simulink model "Foc"  (R2025b)
settings: Solver=FixedStepDiscrete  StartTime=0.0  StopTime=10.0  FixedStep=0.001  RelTol=1e-3
values from neighbouring files (symbols this model uses):
  cal_bActHwMode = NoneSAR.Parameter    [Foc_2024b_LoadCalParameter.m]    (also in Foc_LoadCalParameter.m)
  cal_f32AdcMaxCountsHw = NoneSAR.Parameter    [Foc_LoadCalParameter.m]
  cal_f32AdcRefVoltHw = NoneSAR.Parameter    [Foc_LoadCalParameter.m]
  cal_f32AdcVoltMidHw = NoneSAR.Parameter    [Foc_LoadCalParameter.m]
  cal_f32FullScaleCur = NoneSAR.Parameter    [Foc_LoadCalParameter.m]
  cal_f32GainAmpHw = NoneSAR.Parameter    [Foc_LoadCalParameter.m]
  cal_f32OhmRShuntHw = NoneSAR.Parameter    [Foc_LoadCalParameter.m]
  cal_s16HwtDutyU = NoneSAR.Parameter    [Foc_LoadCalParameter.m]
  cal_s16HwtDutyV = NoneSAR.Parameter    [Foc_LoadCalParameter.m]
  cal_s16HwtDutyW = NoneSAR.Parameter    [Foc_LoadCalParameter.m]
  cal_s16IdKi = NoneSAR.Parameter    [Foc_LoadCalParameter.m]
  cal_s16IdKp = NoneSAR.Parameter    [Foc_LoadCalParameter.m]
  cal_s16IdMaxOut = NoneSAR.Parameter    [Foc_LoadCalParameter.m]
  cal_s16IdMinOut = NoneSAR.Parameter    [Foc_LoadCalParameter.m]
  cal_s16Inductivity = NoneSAR.Parameter    [Foc_2024b_LoadCalParameter.m]    (also in Foc_LoadCalParameter.m)
  cal_s16IqKi = NoneSAR.Parameter    [Foc_LoadCalParameter.m]
  cal_s16IqKp = NoneSAR.Parameter    [Foc_LoadCalParameter.m]
  cal_s16IqMaxOut = NoneSAR.Parameter    [Foc_LoadCalParameter.m]
  cal_s16IqMinOut = NoneSAR.Parameter    [Foc_LoadCalParameter.m]
  cal_s16LpfPllEst = NoneSAR.Parameter    [Foc_2024b_LoadCalParameter.m]    (also in Foc_LoadCalParameter.m)
  cal_s16LpfPllEstOpenLoop = NoneSAR.Parameter    [Foc_2024b_LoadCalParameter.m]    (also in Foc_LoadCalParameter.m)
  cal_s16MinSampleTime = NoneSAR.Parameter    [Foc_2024b_LoadCalParameter.m]    (also in Foc_LoadCalParameter.m)
  cal_s16OmegaGainEst = NoneSAR.Parameter    [Foc_2024b_LoadCalParameter.m]    (also in Foc_LoadCalParameter.m)
  cal_s16RPha = NoneSAR.Parameter    [Foc_2024b_LoadCalParameter.m]    (also in Foc_LoadCalParameter.m)
  cal_s16ThresholdPhaCurImplaisible = NoneSAR.Parameter    [Foc_2024b_LoadCalParameter.m]    (also in Foc_LoadCalParameter.m)
  cal_s8IdFacKi = NoneSAR.Parameter    [Foc_LoadCalParameter.m]
  cal_s8IdFacKp = NoneSAR.Parameter    [Foc_LoadCalParameter.m]
  cal_s8IqFacKi = NoneSAR.Parameter    [Foc_LoadCalParameter.m]
  cal_s8IqFacKp = NoneSAR.Parameter    [Foc_LoadCalParameter.m]
  cal_u16AdcTriggerOffset = NoneSAR.Parameter    [Foc_LoadCalParameter.m]
  cal_u8HwtSector = NoneSAR.Parameter    [Foc_LoadCalParameter.m]
  cal_u8TiDebPhaCur = NoneSAR.Parameter    [Foc_2024b_LoadCalParameter.m]    (also in Foc_LoadCalParameter.m)
undefined symbols (not defined in the file or in its folder): CCU6_T12PERIOD, CCU_PWM_PERIOD_TICKS_HALF, DCLINK_VOLTAGE_FACTOR, DesiredPwm_U, DesiredPwm_V, DesiredPwm_W, e_motorstate_t, e_running_dir_t, FOC_SVM_MAX, FOC_VD_VQ_MAX, FOC_VD_VQ_MAX_100, FOC_VD_VQ_MAX_95, FOC_VD_VQ_MAX_97, FOCLLD_CCU_PWM_PERIOD_TICKS_HALF, FOCLLD_SKIP_DEAD_TIME_THRESHOLD, MAX_DUTY, MIN_SAMPLE_TIME_DEFAULT, MODULATION_FLATBOTTOM, ONEBY_CURRENT_AMPLIFICATION, PhaseCurrentU, PhaseCurrentV, PhaseCurrentW, PwmShift_DutyLong, PwmShift_DutyMed, PwmShift_DutyShort, PwmShiftPtr_RiseLong, PwmShiftPtr_RiseMed, PwmShiftPtr_RiseShort, s16_EST_THETA_GAIN, s16_ONEBYSQR3, s16_SQR3OVER2, st_c_pi_Q_s16_outMax, st_c_pi_Q_s16_outMin, U8_INDUCTIVITY_FAC, VQ_MAX_TABLE_SIZE, VqMaxTable_100, VqMaxTable_95, VqMaxTable_97
libraries: simulink x16, hdlsllib x2
(part 5 of 6)

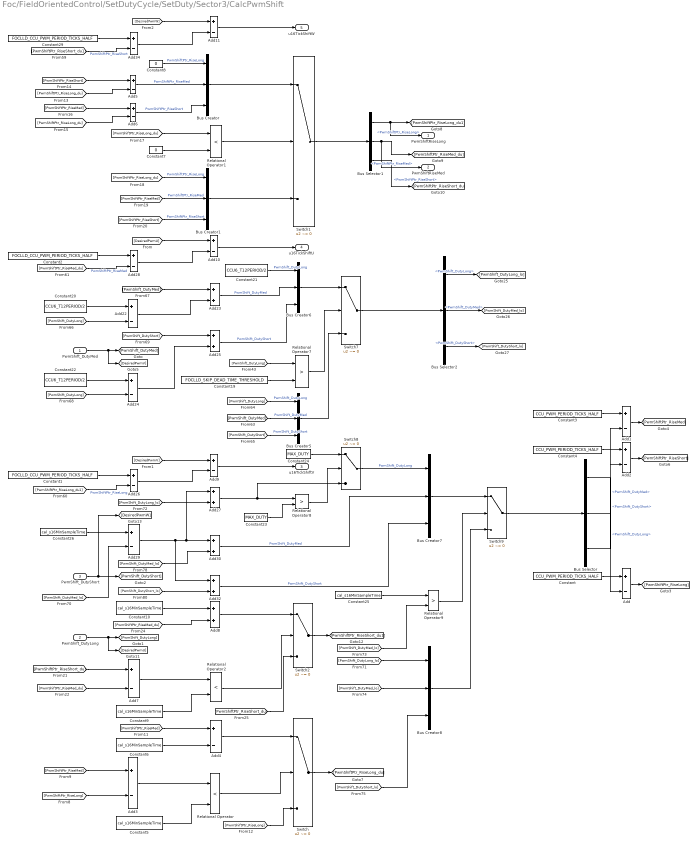
== system Foc/FieldOrientedControl/SetDutyCycle/SetDuty/Sector3/CalcPwmShift ==
  PwmShift_DutyMed : Inport
  PwmShift_DutyLong : Inport  Port=2
  PwmShift_DutyShort : Inport  Port=3
  Add{,1..7,9..11,22,24,26,28..29,34} (17 alike) : Sum  Inputs=+-
  Add{8,23,25,27,30,32} (6 alike) : Sum
  Bus Creator : BusCreator  Inputs=PwmShiftPtr_RiseLong,PwmShiftPtr_RiseMed,PwmShiftPtr_RiseShort
  Bus Creator1 : BusCreator  Inputs=PwmShiftPtr_RiseLong,PwmShiftPtr_RiseMed,PwmShiftPtr_RiseShort
  Bus Creator{5..8} (4 alike) : BusCreator  Inputs=PwmShift_DutyLong,PwmShift_DutyMed,PwmShift_DutyShort
  Bus Selector : BusSelector  OutputSignals=PwmShift_DutyLong,PwmShift_DutyMed,PwmShift_DutyShort
  Bus Selector1 : BusSelector  OutputSignals=PwmShiftPtr_RiseLong,PwmShiftPtr_RiseMed,PwmShiftPtr_RiseShort
  Bus Selector2 : BusSelector  OutputSignals=PwmShift_DutyLong,PwmShift_DutyMed,PwmShift_DutyShort
  Constant : Constant  Value=CCU_PWM_PERIOD_TICKS_HALF
  Constant1 : Constant  Value=FOCLLD_CCU_PWM_PERIOD_TICKS_HALF
  Constant{5..6,9..10,25..26} (6 alike) : Constant  Value=cal_s16MinSampleTime
  Constant19 : Constant  Value=FOCLLD_SKIP_DEAD_TIME_THRESHOLD
  Constant2 : Constant  Value=FOCLLD_CCU_PWM_PERIOD_TICKS_HALF
  Constant20 : Constant  Value=CCU6_T12PERIOD/2
  Constant21 : Constant  Value=CCU6_T12PERIOD/2
  Constant22 : Constant  Value=CCU6_T12PERIOD/2
  Constant23 : Constant  Value=MAX_DUTY
  Constant24 : Constant  Value=MAX_DUTY
  Constant29 : Constant  Value=FOCLLD_CCU_PWM_PERIOD_TICKS_HALF
  Constant3 : Constant  Value=CCU_PWM_PERIOD_TICKS_HALF
  Constant4 : Constant  Value=CCU_PWM_PERIOD_TICKS_HALF
  Constant7 : Constant  Value=0  OutDataTypeStr=int16
  Constant8 : Constant  Value=0  OutDataTypeStr=int16
  Relational Operator : RelationalOperator  Operator=<  OutDataTypeStr=boolean  RndMeth=Simplest  InputSameDT=off
  Relational Operator1 : RelationalOperator  Operator=<  OutDataTypeStr=boolean  RndMeth=Simplest  InputSameDT=off
  Relational Operator2 : RelationalOperator  Operator=<  OutDataTypeStr=boolean  RndMeth=Simplest  InputSameDT=off
  Relational Operator7 : RelationalOperator  Operator=>  OutDataTypeStr=boolean  RndMeth=Simplest  InputSameDT=off
  Relational Operator8 : RelationalOperator  Operator=>  OutDataTypeStr=boolean  RndMeth=Simplest  InputSameDT=off
  Relational Operator9 : RelationalOperator  Operator=>  OutDataTypeStr=boolean  RndMeth=Simplest  InputSameDT=off
  Switch{,1..2,7..9} (6 alike) : Switch  Criteria=u2 ~= 0  SaturateOnIntegerOverflow=off  InputSameDT=off
  PwmShiftRiseLong : Outport
  PwmShiftRiseMed : Outport  Port=2
  u16TickShiftV : Outport  Port=3  OutDataTypeStr=uint16
  u16TickShiftU : Outport  Port=4  OutDataTypeStr=uint16
  u16TickShiftW : Outport  Port=5  OutDataTypeStr=uint16
  wires:
  Constant2/1 -> Add28/1
  [PwmShiftPtr_RiseLong_du] -> Add5/2
  Constant29/1 -> Add34/1
  [PwmShiftPtr_RiseShort_du1] -> Add34/2  "PwmShiftPtr_RiseShort"
  Bus Creator/1 -> Switch1/1
  [PwmShiftPtr_RiseShort] -> Add5/1
  [PwmShiftPtr_RiseMed] -> Add6/1
  [PwmShiftPtr_RiseLong_du] -> Add6/2
  [PwmShiftPtr_RiseMed_du] -> Add28/2  "PwmShiftPtr_RiseMed"
  Constant20/1 -> Add22/1
  [PwmShift_DutyLong] -> Add22/2
  PwmShift_DutyMed/1 -> [DesiredPwmV], [PwmShift_DutyMed]
  Constant22/1 -> Add24/1
  Relational Operator1/1 -> Switch1/2
  [PwmShift_DutyLong] -> Add24/2
  Constant1/1 -> Add26/1
  [PwmShiftPtr_RiseLong_du1] -> Add26/2  "PwmShiftPtr_RiseLong"
  Add7/1 -> Relational Operator2/1
  Constant26/1 -> Add29/1
  PwmShift_DutyShort/1 -> [DesiredPwmW], [PwmShift_DutyShort]
  Bus Creator7/1 -> Switch9/1
  [PwmShift_DutyMed_lo] -> Add29/2
  PwmShift_DutyLong/1 -> [DesiredPwmU], [PwmShift_DutyLong]
  Add22/1 -> Add23/2
  Add8/1 -> Switch2/1
  [PwmShiftPtr_RiseShort_du] -> Add7/1
  [PwmShiftPtr_RiseMed_du] -> Add7/2
  Bus Selector2/2 -> [PwmShift_DutyMed_lo]  "<PwmShift_DutyMed>"
  [PwmShiftPtr_RiseMed] -> Add3/1
  Add29/1 -> Add30/1, Add27/1, Add32/1
  [PwmShiftPtr_RiseLong] -> Add3/2
  [DesiredPwmW] -> Add11/1
  Add34/1 -> Add11/2
  Constant8/1 -> Bus Creator/1  "PwmShiftPtr_RiseLong"
  Add10/1 -> u16TickShiftU/1
  Add5/1 -> Bus Creator/2  "PwmShiftPtr_RiseMed"
  [PwmShiftPtr_RiseMed_du] -> Add8/2
  Add11/1 -> u16TickShiftW/1
  Add6/1 -> Bus Creator/3  "PwmShiftPtr_RiseShort"
  [PwmShiftPtr_RiseLong_du] -> Relational Operator1/1
  Constant7/1 -> Relational Operator1/2
  [PwmShiftPtr_RiseLong_du] -> Bus Creator1/1  "PwmShiftPtr_RiseLong"
  [PwmShiftPtr_RiseMed] -> Bus Creator1/2  "PwmShiftPtr_RiseMed"
  [PwmShiftPtr_RiseShort] -> Bus Creator1/3  "PwmShiftPtr_RiseShort"
  [DesiredPwmU] -> Add10/1
  [PwmShift_DutyMed] -> Add23/1
  Add28/1 -> Add10/2
  Add25/1 -> Bus Creator6/3  "PwmShift_DutyShort"
  [PwmShift_DutyShort] -> Add25/1
  [PwmShift_DutyLong] -> Relational Operator7/1
  Add24/1 -> Add25/2
  [DesiredPwmV] -> Add9/1
  Add26/1 -> Add9/2
  [PwmShift_DutyLong_lo] -> Add27/2
  Bus Selector1/1 -> PwmShiftRiseLong/1, [PwmShiftPtr_RiseLong_du1]  "<PwmShiftPtr_RiseLong>"
  [PwmShift_DutyMed_lo] -> Add30/2
  [PwmShift_DutyShort_lo] -> Add32/2
  Constant10/1 -> Add8/1
  Constant9/1 -> Relational Operator2/2
  [PwmShiftPtr_RiseMed] -> Add4/1
  Constant6/1 -> Add4/2
  Add3/1 -> Relational Operator/1
  Constant5/1 -> Relational Operator/2
  Bus Creator1/1 -> Switch1/3
  Constant21/1 -> Bus Creator6/1  "PwmShift_DutyLong"
  Add23/1 -> Bus Creator6/2  "PwmShift_DutyMed"
  Constant19/1 -> Relational Operator7/2
  [PwmShift_DutyLong] -> Bus Creator5/1  "PwmShift_DutyLong"
  [PwmShift_DutyMed] -> Bus Creator5/2  "PwmShift_DutyMed"
  Add9/1 -> u16TickShiftV/1
  [PwmShift_DutyShort] -> Bus Creator5/3  "PwmShift_DutyShort"
  Add27/1 -> Switch8/3, Relational Operator8/1
  Constant23/1 -> Relational Operator8/2
  Add30/1 -> Bus Creator7/2  "PwmShift_DutyMed"
  Add32/1 -> Bus Creator7/3  "PwmShift_DutyShort"
  Relational Operator2/1 -> Switch2/2
  [PwmShiftPtr_RiseShort_du] -> Switch2/3
  Add4/1 -> Switch/1
  Relational Operator/1 -> Switch/2
  [PwmShiftPtr_RiseLong] -> Switch/3
  Switch1/1 -> Bus Selector1/1
  Bus Creator6/1 -> Switch7/1
  Relational Operator7/1 -> Switch7/2
  [PwmShift_DutyMed_lo] -> Relational Operator9/2
  Bus Creator5/1 -> Switch7/3
  Constant24/1 -> Switch8/1
  Relational Operator8/1 -> Switch8/2
  Switch2/1 -> [PwmShiftPtr_RiseShort_du1]
  Switch/1 -> [PwmShiftPtr_RiseLong_du]
  Bus Selector1/2 -> PwmShiftRiseMed/1, [PwmShiftPtr_RiseMed_du]  "<PwmShiftPtr_RiseMed>"
  Bus Selector1/3 -> [PwmShiftPtr_RiseShort_du]  "<PwmShiftPtr_RiseShort>"
  Switch7/1 -> Bus Selector2/1
  Switch8/1 -> Bus Creator7/1  "PwmShift_DutyLong"
  Constant25/1 -> Relational Operator9/1
  [PwmShift_DutyLong_lo] -> Bus Creator8/1
  Bus Selector/2 -> Add1/2  "<PwmShift_DutyMed>"
  [PwmShift_DutyMed_lo] -> Bus Creator8/2
  [PwmShift_DutyShort_lo] -> Bus Creator8/3
  Bus Selector2/1 -> [PwmShift_DutyLong_lo]  "<PwmShift_DutyLong>"
  Bus Selector2/3 -> [PwmShift_DutyShort_lo]  "<PwmShift_DutyShort>"
  Relational Operator9/1 -> Switch9/2
  Bus Creator8/1 -> Switch9/3
  Switch9/1 -> Bus Selector/1
  Constant3/1 -> Add1/1
  Constant4/1 -> Add2/1
  Bus Selector/1 -> Add/2  "<PwmShift_DutyLong>"
  Bus Selector/3 -> Add2/2  "<PwmShift_DutyShort>"
  Constant/1 -> Add/1
  Add1/1 -> [PwmShiftPtr_RiseMed]
  Add2/1 -> [PwmShiftPtr_RiseShort]
  Add/1 -> [PwmShiftPtr_RiseLong]

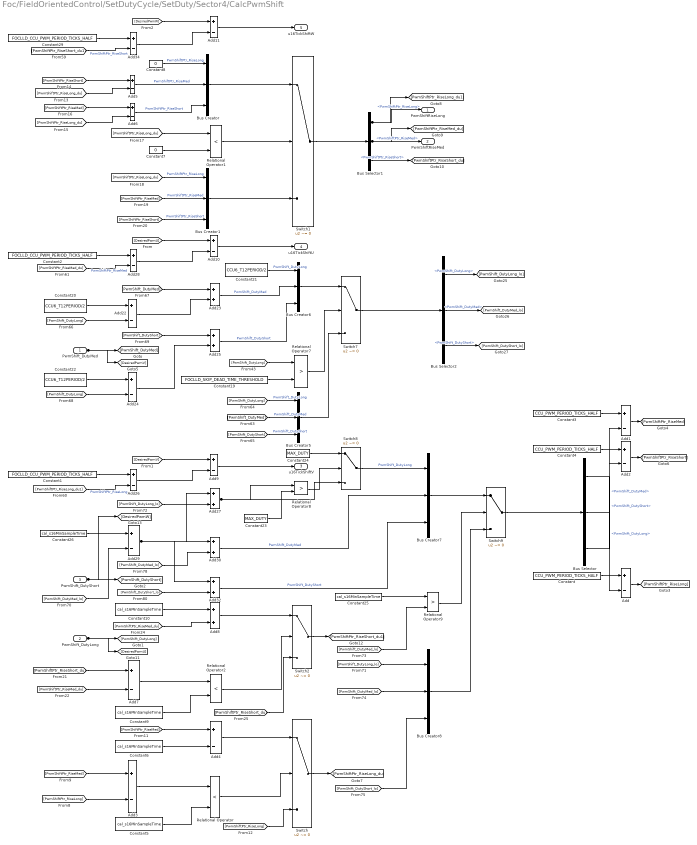
== system Foc/FieldOrientedControl/SetDutyCycle/SetDuty/Sector4/CalcPwmShift ==
  PwmShift_DutyMed : Inport
  PwmShift_DutyLong : Inport  Port=2
  PwmShift_DutyShort : Inport  Port=3
  Add{,1..7,9..11,22,24,26,28..29,34} (17 alike) : Sum  Inputs=+-
  Add{8,23,25,27,30,32} (6 alike) : Sum
  Bus Creator : BusCreator  Inputs=PwmShiftPtr_RiseLong,PwmShiftPtr_RiseMed,PwmShiftPtr_RiseShort
  Bus Creator1 : BusCreator  Inputs=PwmShiftPtr_RiseLong,PwmShiftPtr_RiseMed,PwmShiftPtr_RiseShort
  Bus Creator{5..8} (4 alike) : BusCreator  Inputs=PwmShift_DutyLong,PwmShift_DutyMed,PwmShift_DutyShort
  Bus Selector : BusSelector  OutputSignals=PwmShift_DutyLong,PwmShift_DutyMed,PwmShift_DutyShort
  Bus Selector1 : BusSelector  OutputSignals=PwmShiftPtr_RiseLong,PwmShiftPtr_RiseMed,PwmShiftPtr_RiseShort
  Bus Selector2 : BusSelector  OutputSignals=PwmShift_DutyLong,PwmShift_DutyMed,PwmShift_DutyShort
  Constant : Constant  Value=CCU_PWM_PERIOD_TICKS_HALF
  Constant1 : Constant  Value=FOCLLD_CCU_PWM_PERIOD_TICKS_HALF
  Constant{5..6,9..10,25..26} (6 alike) : Constant  Value=cal_s16MinSampleTime
  Constant19 : Constant  Value=FOCLLD_SKIP_DEAD_TIME_THRESHOLD
  Constant2 : Constant  Value=FOCLLD_CCU_PWM_PERIOD_TICKS_HALF
  Constant20 : Constant  Value=CCU6_T12PERIOD/2
  Constant21 : Constant  Value=CCU6_T12PERIOD/2
  Constant22 : Constant  Value=CCU6_T12PERIOD/2
  Constant23 : Constant  Value=MAX_DUTY
  Constant24 : Constant  Value=MAX_DUTY
  Constant29 : Constant  Value=FOCLLD_CCU_PWM_PERIOD_TICKS_HALF
  Constant3 : Constant  Value=CCU_PWM_PERIOD_TICKS_HALF
  Constant4 : Constant  Value=CCU_PWM_PERIOD_TICKS_HALF
  Constant7 : Constant  Value=0  OutDataTypeStr=int16
  Constant8 : Constant  Value=0  OutDataTypeStr=int16
  Relational Operator : RelationalOperator  Operator=<  OutDataTypeStr=boolean  RndMeth=Simplest  InputSameDT=off
  Relational Operator1 : RelationalOperator  Operator=<  OutDataTypeStr=boolean  RndMeth=Simplest  InputSameDT=off
  Relational Operator2 : RelationalOperator  Operator=<  OutDataTypeStr=boolean  RndMeth=Simplest  InputSameDT=off
  Relational Operator7 : RelationalOperator  Operator=>  OutDataTypeStr=boolean  RndMeth=Simplest  InputSameDT=off
  Relational Operator8 : RelationalOperator  Operator=>  OutDataTypeStr=boolean  RndMeth=Simplest  InputSameDT=off
  Relational Operator9 : RelationalOperator  Operator=>  OutDataTypeStr=boolean  RndMeth=Simplest  InputSameDT=off
  Switch{,1..2,7..9} (6 alike) : Switch  Criteria=u2 ~= 0  SaturateOnIntegerOverflow=off  InputSameDT=off
  PwmShiftRiseLong : Outport
  PwmShiftRiseMed : Outport  Port=2
  u16TickShiftV : Outport  Port=3  OutDataTypeStr=uint16
  u16TickShiftU : Outport  Port=4  OutDataTypeStr=uint16
  u16TickShiftW : Outport  Port=5  OutDataTypeStr=uint16
  wires:
  Constant2/1 -> Add28/1
  [PwmShiftPtr_RiseLong_du] -> Add5/2
  Constant29/1 -> Add34/1
  [PwmShiftPtr_RiseLong_du] -> Add6/2
  [PwmShiftPtr_RiseShort_du1] -> Add34/2  "PwmShiftPtr_RiseShort"
  Bus Creator/1 -> Switch1/1
  [PwmShiftPtr_RiseShort] -> Add5/1
  Add10/1 -> u16TickShiftU/1
  [PwmShiftPtr_RiseMed] -> Add6/1
  Add5/1 -> Bus Creator/2  "PwmShiftPtr_RiseMed"
  [PwmShiftPtr_RiseMed_du] -> Add28/2  "PwmShiftPtr_RiseMed"
  Constant20/1 -> Add22/1
  [PwmShift_DutyLong] -> Add22/2
  PwmShift_DutyMed/1 -> [DesiredPwmV], [PwmShift_DutyMed]
  Constant22/1 -> Add24/1
  Relational Operator1/1 -> Switch1/2
  [PwmShift_DutyLong] -> Add24/2
  Constant1/1 -> Add26/1
  Add25/1 -> Bus Creator6/3  "PwmShift_DutyShort"
  [PwmShiftPtr_RiseLong_du1] -> Add26/2  "PwmShiftPtr_RiseLong"
  Constant26/1 -> Add29/1
  Add32/1 -> Bus Creator7/3  "PwmShift_DutyShort"
  [PwmShiftPtr_RiseLong_du] -> Bus Creator1/1  "PwmShiftPtr_RiseLong"
  PwmShift_DutyShort/1 -> [DesiredPwmW], [PwmShift_DutyShort]
  Bus Creator7/1 -> Switch9/1
  [PwmShift_DutyMed_lo] -> Add29/2
  PwmShift_DutyLong/1 -> [DesiredPwmU], [PwmShift_DutyLong]
  Add4/1 -> Switch/1
  [PwmShiftPtr_RiseShort_du] -> Add7/1
  [PwmShiftPtr_RiseMed_du] -> Add7/2
  Add3/1 -> Relational Operator/1
  [PwmShiftPtr_RiseMed] -> Add3/1
  Add34/1 -> Add11/2
  Bus Selector1/3 -> [PwmShiftPtr_RiseShort_du]  "<PwmShiftPtr_RiseShort>"
  [PwmShiftPtr_RiseLong] -> Add3/2
  [DesiredPwmW] -> Add11/1
  Add7/1 -> Relational Operator2/1
  Constant8/1 -> Bus Creator/1  "PwmShiftPtr_RiseLong"
  Add6/1 -> Bus Creator/3  "PwmShiftPtr_RiseShort"
  [PwmShift_DutyLong] -> Relational Operator7/1
  Add11/1 -> u16TickShiftW/1
  [PwmShiftPtr_RiseLong_du] -> Relational Operator1/1
  Constant7/1 -> Relational Operator1/2
  [PwmShiftPtr_RiseMed] -> Bus Creator1/2  "PwmShiftPtr_RiseMed"
  [PwmShiftPtr_RiseShort] -> Bus Creator1/3  "PwmShiftPtr_RiseShort"
  [DesiredPwmU] -> Add10/1
  Add28/1 -> Add10/2
  Add24/1 -> Add25/2
  [PwmShift_DutyMed] -> Add23/1
  Add22/1 -> Add23/2
  Add29/1 -> Add32/1, Add30/1, Add27/1
  [PwmShift_DutyShort] -> Add25/1
  [DesiredPwmV] -> Add9/1
  Add26/1 -> Add9/2
  [PwmShift_DutyLong_lo] -> Add27/2
  Bus Selector1/1 -> PwmShiftRiseLong/1, [PwmShiftPtr_RiseLong_du1]  "<PwmShiftPtr_RiseLong>"
  [PwmShift_DutyMed_lo] -> Add30/2
  [PwmShift_DutyShort_lo] -> Add32/2
  Constant10/1 -> Add8/1
  Add23/1 -> Bus Creator6/2  "PwmShift_DutyMed"
  Add9/1 -> u16TickShiftV/1
  [PwmShiftPtr_RiseMed_du] -> Add8/2
  Constant9/1 -> Relational Operator2/2
  [PwmShiftPtr_RiseMed] -> Add4/1
  Constant6/1 -> Add4/2
  Constant5/1 -> Relational Operator/2
  Bus Creator1/1 -> Switch1/3
  Constant21/1 -> Bus Creator6/1  "PwmShift_DutyLong"
  Constant19/1 -> Relational Operator7/2
  [PwmShift_DutyLong] -> Bus Creator5/1  "PwmShift_DutyLong"
  Add8/1 -> Switch2/1
  [PwmShift_DutyMed] -> Bus Creator5/2  "PwmShift_DutyMed"
  Bus Creator5/1 -> Switch7/3
  [PwmShift_DutyShort] -> Bus Creator5/3  "PwmShift_DutyShort"
  Add27/1 -> Switch8/3, Relational Operator8/1
  Constant23/1 -> Relational Operator8/2
  Add30/1 -> Bus Creator7/2  "PwmShift_DutyMed"
  Relational Operator2/1 -> Switch2/2
  [PwmShiftPtr_RiseShort_du] -> Switch2/3
  Relational Operator/1 -> Switch/2
  [PwmShiftPtr_RiseLong] -> Switch/3
  Switch1/1 -> Bus Selector1/1
  Bus Creator6/1 -> Switch7/1
  Relational Operator7/1 -> Switch7/2
  Constant24/1 -> Switch8/1
  Relational Operator8/1 -> Switch8/2
  Switch2/1 -> [PwmShiftPtr_RiseShort_du1]
  Switch/1 -> [PwmShiftPtr_RiseLong_du]
  Bus Selector1/2 -> PwmShiftRiseMed/1, [PwmShiftPtr_RiseMed_du]  "<PwmShiftPtr_RiseMed>"
  Switch7/1 -> Bus Selector2/1
  Switch8/1 -> Bus Creator7/1  "PwmShift_DutyLong"
  Constant25/1 -> Relational Operator9/1
  [PwmShift_DutyMed_lo] -> Relational Operator9/2
  [PwmShift_DutyLong_lo] -> Bus Creator8/1
  Bus Selector/2 -> Add1/2  "<PwmShift_DutyMed>"
  [PwmShift_DutyMed_lo] -> Bus Creator8/2
  [PwmShift_DutyShort_lo] -> Bus Creator8/3
  Bus Selector2/1 -> [PwmShift_DutyLong_lo]  "<PwmShift_DutyLong>"
  Bus Selector2/2 -> [PwmShift_DutyMed_lo]  "<PwmShift_DutyMed>"
  Bus Selector2/3 -> [PwmShift_DutyShort_lo]  "<PwmShift_DutyShort>"
  Relational Operator9/1 -> Switch9/2
  Bus Creator8/1 -> Switch9/3
  Switch9/1 -> Bus Selector/1
  Constant3/1 -> Add1/1
  Constant4/1 -> Add2/1
  Bus Selector/1 -> Add/2  "<PwmShift_DutyLong>"
  Bus Selector/3 -> Add2/2  "<PwmShift_DutyShort>"
  Constant/1 -> Add/1
  Add1/1 -> [PwmShiftPtr_RiseMed]
  Add2/1 -> [PwmShiftPtr_RiseShort]
  Add/1 -> [PwmShiftPtr_RiseLong]

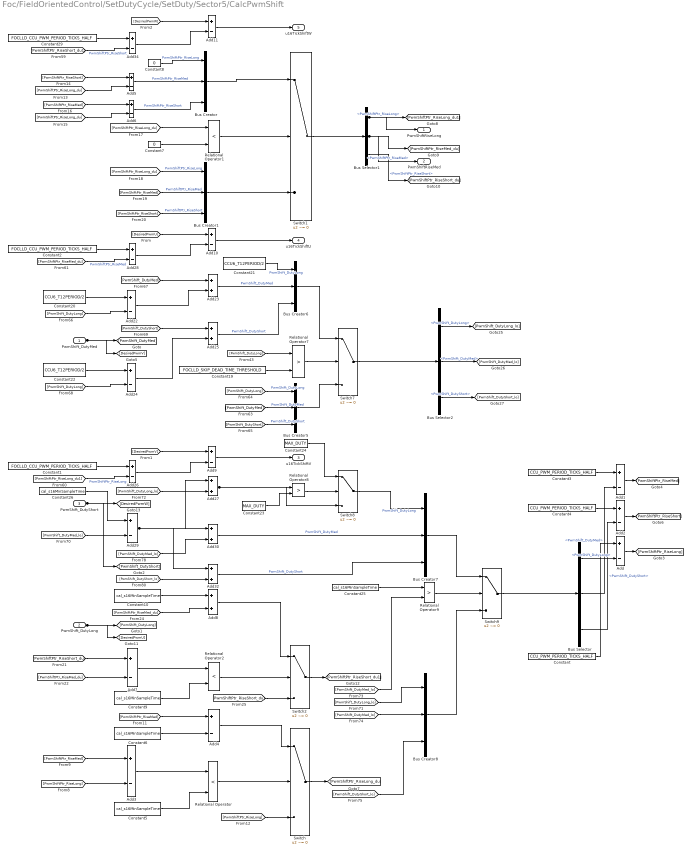
== system Foc/FieldOrientedControl/SetDutyCycle/SetDuty/Sector5/CalcPwmShift ==
  PwmShift_DutyMed : Inport
  PwmShift_DutyLong : Inport  Port=2
  PwmShift_DutyShort : Inport  Port=3
  Add{,1..7,9..11,22,24,26,28..29,34} (17 alike) : Sum  Inputs=+-
  Add{8,23,25,27,30,32} (6 alike) : Sum
  Bus Creator : BusCreator  Inputs=PwmShiftPtr_RiseLong,PwmShiftPtr_RiseMed,PwmShiftPtr_RiseShort
  Bus Creator1 : BusCreator  Inputs=PwmShiftPtr_RiseLong,PwmShiftPtr_RiseMed,PwmShiftPtr_RiseShort
  Bus Creator{5..8} (4 alike) : BusCreator  Inputs=PwmShift_DutyLong,PwmShift_DutyMed,PwmShift_DutyShort
  Bus Selector : BusSelector  OutputSignals=PwmShift_DutyLong,PwmShift_DutyMed,PwmShift_DutyShort
  Bus Selector1 : BusSelector  OutputSignals=PwmShiftPtr_RiseLong,PwmShiftPtr_RiseMed,PwmShiftPtr_RiseShort
  Bus Selector2 : BusSelector  OutputSignals=PwmShift_DutyLong,PwmShift_DutyMed,PwmShift_DutyShort
  Constant : Constant  Value=CCU_PWM_PERIOD_TICKS_HALF
  Constant1 : Constant  Value=FOCLLD_CCU_PWM_PERIOD_TICKS_HALF
  Constant{5..6,9..10,25..26} (6 alike) : Constant  Value=cal_s16MinSampleTime
  Constant19 : Constant  Value=FOCLLD_SKIP_DEAD_TIME_THRESHOLD
  Constant2 : Constant  Value=FOCLLD_CCU_PWM_PERIOD_TICKS_HALF
  Constant20 : Constant  Value=CCU6_T12PERIOD/2
  Constant21 : Constant  Value=CCU6_T12PERIOD/2
  Constant22 : Constant  Value=CCU6_T12PERIOD/2
  Constant23 : Constant  Value=MAX_DUTY
  Constant24 : Constant  Value=MAX_DUTY
  Constant29 : Constant  Value=FOCLLD_CCU_PWM_PERIOD_TICKS_HALF
  Constant3 : Constant  Value=CCU_PWM_PERIOD_TICKS_HALF
  Constant4 : Constant  Value=CCU_PWM_PERIOD_TICKS_HALF
  Constant7 : Constant  Value=0  OutDataTypeStr=int16
  Constant8 : Constant  Value=0  OutDataTypeStr=int16
  Relational Operator : RelationalOperator  Operator=<  OutDataTypeStr=boolean  RndMeth=Simplest  InputSameDT=off
  Relational Operator1 : RelationalOperator  Operator=<  OutDataTypeStr=boolean  RndMeth=Simplest  InputSameDT=off
  Relational Operator2 : RelationalOperator  Operator=<  OutDataTypeStr=boolean  RndMeth=Simplest  InputSameDT=off
  Relational Operator7 : RelationalOperator  Operator=>  OutDataTypeStr=boolean  RndMeth=Simplest  InputSameDT=off
  Relational Operator8 : RelationalOperator  Operator=>  OutDataTypeStr=boolean  RndMeth=Simplest  InputSameDT=off
  Relational Operator9 : RelationalOperator  Operator=>  OutDataTypeStr=boolean  RndMeth=Simplest  InputSameDT=off
  Switch{,1..2,7..9} (6 alike) : Switch  Criteria=u2 ~= 0  SaturateOnIntegerOverflow=off  InputSameDT=off
  PwmShiftRiseLong : Outport
  PwmShiftRiseMed : Outport  Port=2
  u16TickShiftV : Outport  Port=3  OutDataTypeStr=uint16
  u16TickShiftU : Outport  Port=4  OutDataTypeStr=uint16
  u16TickShiftW : Outport  Port=5  OutDataTypeStr=uint16
  wires:
  Constant2/1 -> Add28/1
  Constant29/1 -> Add34/1
  [PwmShiftPtr_RiseLong_du] -> Add6/2
  [PwmShiftPtr_RiseShort_du1] -> Add34/2  "PwmShiftPtr_RiseShort"
  Bus Creator/1 -> Switch1/1
  Bus Selector2/2 -> [PwmShift_DutyMed_lo]  "<PwmShift_DutyMed>"
  [PwmShiftPtr_RiseMed] -> Add3/1
  Add4/1 -> Switch/1
  [PwmShiftPtr_RiseShort] -> Add5/1
  [PwmShiftPtr_RiseMed_du] -> Add28/2  "PwmShiftPtr_RiseMed"
  [PwmShift_DutyShort_lo] -> Add32/2
  [PwmShiftPtr_RiseLong_du] -> Add5/2
  PwmShift_DutyMed/1 -> [DesiredPwmV], [PwmShift_DutyMed]
  Add30/1 -> Bus Creator7/2  "PwmShift_DutyMed"
  [PwmShiftPtr_RiseMed] -> Add6/1
  Constant20/1 -> Add22/1
  [PwmShift_DutyLong] -> Add22/2
  Constant22/1 -> Add24/1
  Relational Operator1/1 -> Switch1/2
  [PwmShift_DutyLong] -> Add24/2
  Constant1/1 -> Add26/1
  [PwmShiftPtr_RiseLong_du1] -> Add26/2  "PwmShiftPtr_RiseLong"
  Add7/1 -> Relational Operator2/1
  Constant26/1 -> Add29/1
  Add32/1 -> Bus Creator7/3  "PwmShift_DutyShort"
  [DesiredPwmV] -> Add9/1
  PwmShift_DutyShort/1 -> [DesiredPwmW], [PwmShift_DutyShort]
  Bus Creator7/1 -> Switch9/1
  [PwmShift_DutyMed_lo] -> Add29/2
  [DesiredPwmU] -> Add10/1
  PwmShift_DutyLong/1 -> [DesiredPwmU], [PwmShift_DutyLong]
  Add22/1 -> Add23/2
  Add8/1 -> Switch2/1
  [PwmShiftPtr_RiseShort_du] -> Add7/1
  [PwmShiftPtr_RiseMed_du] -> Add7/2
  [PwmShiftPtr_RiseLong] -> Switch/3
  Add29/1 -> Add30/1, Add32/1, Add27/1
  [PwmShiftPtr_RiseLong] -> Add3/2
  [DesiredPwmW] -> Add11/1
  Add34/1 -> Add11/2
  Constant8/1 -> Bus Creator/1  "PwmShiftPtr_RiseLong"
  Add10/1 -> u16TickShiftU/1
  Add5/1 -> Bus Creator/2  "PwmShiftPtr_RiseMed"
  [PwmShiftPtr_RiseMed_du] -> Add8/2
  Add11/1 -> u16TickShiftW/1
  Add6/1 -> Bus Creator/3  "PwmShiftPtr_RiseShort"
  [PwmShiftPtr_RiseLong_du] -> Bus Creator1/1  "PwmShiftPtr_RiseLong"
  [PwmShiftPtr_RiseLong_du] -> Relational Operator1/1
  Constant7/1 -> Relational Operator1/2
  [PwmShiftPtr_RiseMed] -> Bus Creator1/2  "PwmShiftPtr_RiseMed"
  [PwmShiftPtr_RiseShort] -> Bus Creator1/3  "PwmShiftPtr_RiseShort"
  [PwmShift_DutyMed] -> Add23/1
  Add28/1 -> Add10/2
  Add25/1 -> Bus Creator6/3  "PwmShift_DutyShort"
  [PwmShift_DutyShort] -> Add25/1
  [PwmShift_DutyLong] -> Relational Operator7/1
  Add24/1 -> Add25/2
  Add26/1 -> Add9/2
  [PwmShift_DutyLong_lo] -> Add27/2
  [PwmShiftPtr_RiseMed] -> Add4/1
  Bus Selector1/1 -> PwmShiftRiseLong/1, [PwmShiftPtr_RiseLong_du1]  "<PwmShiftPtr_RiseLong>"
  [PwmShift_DutyMed_lo] -> Add30/2
  Constant10/1 -> Add8/1
  Constant9/1 -> Relational Operator2/2
  Constant6/1 -> Add4/2
  Add3/1 -> Relational Operator/1
  Constant5/1 -> Relational Operator/2
  Bus Creator1/1 -> Switch1/3
  Constant21/1 -> Bus Creator6/1  "PwmShift_DutyLong"
  Add23/1 -> Bus Creator6/2  "PwmShift_DutyMed"
  Constant19/1 -> Relational Operator7/2
  [PwmShift_DutyLong] -> Bus Creator5/1  "PwmShift_DutyLong"
  [PwmShift_DutyMed] -> Bus Creator5/2  "PwmShift_DutyMed"
  Add9/1 -> u16TickShiftV/1
  [PwmShift_DutyShort] -> Bus Creator5/3  "PwmShift_DutyShort"
  Add27/1 -> Switch8/3, Relational Operator8/1
  Constant23/1 -> Relational Operator8/2
  Relational Operator2/1 -> Switch2/2
  [PwmShiftPtr_RiseShort_du] -> Switch2/3
  Relational Operator/1 -> Switch/2
  Switch1/1 -> Bus Selector1/1
  Bus Creator6/1 -> Switch7/1
  Relational Operator7/1 -> Switch7/2
  [PwmShift_DutyMed_lo] -> Relational Operator9/2
  Bus Creator5/1 -> Switch7/3
  Constant24/1 -> Switch8/1
  Relational Operator8/1 -> Switch8/2
  Switch2/1 -> [PwmShiftPtr_RiseShort_du1]
  Switch/1 -> [PwmShiftPtr_RiseLong_du]
  Bus Selector1/2 -> PwmShiftRiseMed/1, [PwmShiftPtr_RiseMed_du]  "<PwmShiftPtr_RiseMed>"
  Bus Selector1/3 -> [PwmShiftPtr_RiseShort_du]  "<PwmShiftPtr_RiseShort>"
  Switch7/1 -> Bus Selector2/1
  Switch8/1 -> Bus Creator7/1  "PwmShift_DutyLong"
  Constant25/1 -> Relational Operator9/1
  [PwmShift_DutyLong_lo] -> Bus Creator8/1
  Bus Selector/2 -> Add1/2  "<PwmShift_DutyMed>"
  [PwmShift_DutyMed_lo] -> Bus Creator8/2
  [PwmShift_DutyShort_lo] -> Bus Creator8/3
  Bus Selector2/1 -> [PwmShift_DutyLong_lo]  "<PwmShift_DutyLong>"
  Bus Selector2/3 -> [PwmShift_DutyShort_lo]  "<PwmShift_DutyShort>"
  Relational Operator9/1 -> Switch9/2
  Bus Creator8/1 -> Switch9/3
  Switch9/1 -> Bus Selector/1
  Constant3/1 -> Add1/1
  Constant4/1 -> Add2/1
  Bus Selector/1 -> Add/2  "<PwmShift_DutyLong>"
  Bus Selector/3 -> Add2/2  "<PwmShift_DutyShort>"
  Constant/1 -> Add/1
  Add1/1 -> [PwmShiftPtr_RiseMed]
  Add2/1 -> [PwmShiftPtr_RiseShort]
  Add/1 -> [PwmShiftPtr_RiseLong]

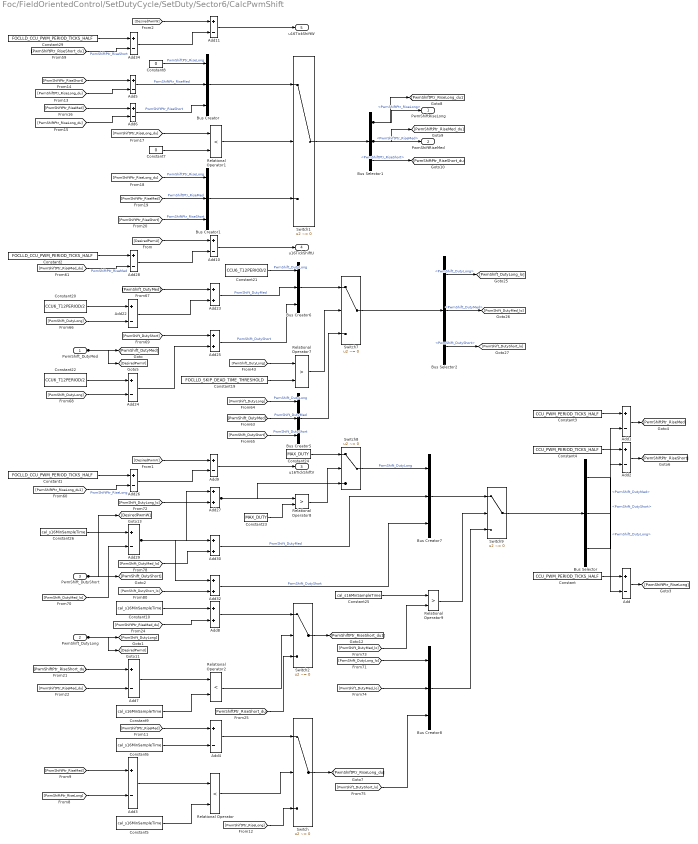
== system Foc/FieldOrientedControl/SetDutyCycle/SetDuty/Sector6/CalcPwmShift ==
  PwmShift_DutyMed : Inport
  PwmShift_DutyLong : Inport  Port=2
  PwmShift_DutyShort : Inport  Port=3
  Add{,1..7,9..11,22,24,26,28..29,34} (17 alike) : Sum  Inputs=+-
  Add{8,23,25,27,30,32} (6 alike) : Sum
  Bus Creator : BusCreator  Inputs=PwmShiftPtr_RiseLong,PwmShiftPtr_RiseMed,PwmShiftPtr_RiseShort
  Bus Creator1 : BusCreator  Inputs=PwmShiftPtr_RiseLong,PwmShiftPtr_RiseMed,PwmShiftPtr_RiseShort
  Bus Creator{5..8} (4 alike) : BusCreator  Inputs=PwmShift_DutyLong,PwmShift_DutyMed,PwmShift_DutyShort
  Bus Selector : BusSelector  OutputSignals=PwmShift_DutyLong,PwmShift_DutyMed,PwmShift_DutyShort
  Bus Selector1 : BusSelector  OutputSignals=PwmShiftPtr_RiseLong,PwmShiftPtr_RiseMed,PwmShiftPtr_RiseShort
  Bus Selector2 : BusSelector  OutputSignals=PwmShift_DutyLong,PwmShift_DutyMed,PwmShift_DutyShort
  Constant : Constant  Value=CCU_PWM_PERIOD_TICKS_HALF
  Constant1 : Constant  Value=FOCLLD_CCU_PWM_PERIOD_TICKS_HALF
  Constant{5..6,9..10,25..26} (6 alike) : Constant  Value=cal_s16MinSampleTime
  Constant19 : Constant  Value=FOCLLD_SKIP_DEAD_TIME_THRESHOLD
  Constant2 : Constant  Value=FOCLLD_CCU_PWM_PERIOD_TICKS_HALF
  Constant20 : Constant  Value=CCU6_T12PERIOD/2
  Constant21 : Constant  Value=CCU6_T12PERIOD/2
  Constant22 : Constant  Value=CCU6_T12PERIOD/2
  Constant23 : Constant  Value=MAX_DUTY
  Constant24 : Constant  Value=MAX_DUTY
  Constant29 : Constant  Value=FOCLLD_CCU_PWM_PERIOD_TICKS_HALF
  Constant3 : Constant  Value=CCU_PWM_PERIOD_TICKS_HALF
  Constant4 : Constant  Value=CCU_PWM_PERIOD_TICKS_HALF
  Constant7 : Constant  Value=0  OutDataTypeStr=int16
  Constant8 : Constant  Value=0  OutDataTypeStr=int16
  Relational Operator : RelationalOperator  Operator=<  OutDataTypeStr=boolean  RndMeth=Simplest  InputSameDT=off
  Relational Operator1 : RelationalOperator  Operator=<  OutDataTypeStr=boolean  RndMeth=Simplest  InputSameDT=off
  Relational Operator2 : RelationalOperator  Operator=<  OutDataTypeStr=boolean  RndMeth=Simplest  InputSameDT=off
  Relational Operator7 : RelationalOperator  Operator=>  OutDataTypeStr=boolean  RndMeth=Simplest  InputSameDT=off
  Relational Operator8 : RelationalOperator  Operator=>  OutDataTypeStr=boolean  RndMeth=Simplest  InputSameDT=off
  Relational Operator9 : RelationalOperator  Operator=>  OutDataTypeStr=boolean  RndMeth=Simplest  InputSameDT=off
  Switch{,1..2,7..9} (6 alike) : Switch  Criteria=u2 ~= 0  SaturateOnIntegerOverflow=off  InputSameDT=off
  PwmShiftRiseLong : Outport
  PwmShiftRiseMed : Outport  Port=2
  u16TickShiftV : Outport  Port=3  OutDataTypeStr=uint16
  u16TickShiftU : Outport  Port=4  OutDataTypeStr=uint16
  u16TickShiftW : Outport  Port=5  OutDataTypeStr=uint16
  wires:
  Constant2/1 -> Add28/1
  Constant29/1 -> Add34/1
  [PwmShiftPtr_RiseLong_du] -> Add6/2
  [PwmShiftPtr_RiseShort_du1] -> Add34/2  "PwmShiftPtr_RiseShort"
  Bus Creator/1 -> Switch1/1
  [PwmShiftPtr_RiseShort] -> Add5/1
  Add3/1 -> Relational Operator/1
  [PwmShiftPtr_RiseMed] -> Add3/1
  [PwmShiftPtr_RiseMed_du] -> Add28/2  "PwmShiftPtr_RiseMed"
  [PwmShift_DutyShort_lo] -> Add32/2
  [PwmShiftPtr_RiseLong_du] -> Add5/2
  Add10/1 -> u16TickShiftU/1
  [PwmShiftPtr_RiseMed] -> Add6/1
  Add5/1 -> Bus Creator/2  "PwmShiftPtr_RiseMed"
  Constant20/1 -> Add22/1
  [PwmShift_DutyLong] -> Add22/2
  Add30/1 -> Bus Creator7/2  "PwmShift_DutyMed"
  Constant9/1 -> Relational Operator2/2
  PwmShift_DutyMed/1 -> [DesiredPwmV], [PwmShift_DutyMed]
  Constant22/1 -> Add24/1
  Relational Operator1/1 -> Switch1/2
  [PwmShift_DutyLong] -> Add24/2
  Constant1/1 -> Add26/1
  Add25/1 -> Bus Creator6/3  "PwmShift_DutyShort"
  [PwmShiftPtr_RiseLong_du1] -> Add26/2  "PwmShiftPtr_RiseLong"
  Constant26/1 -> Add29/1
  Add32/1 -> Bus Creator7/3  "PwmShift_DutyShort"
  [PwmShiftPtr_RiseLong_du] -> Bus Creator1/1  "PwmShiftPtr_RiseLong"
  PwmShift_DutyShort/1 -> [DesiredPwmW], [PwmShift_DutyShort]
  Constant6/1 -> Add4/2
  Bus Creator7/1 -> Switch9/1
  [PwmShift_DutyMed_lo] -> Add29/2
  [DesiredPwmU] -> Add10/1
  PwmShift_DutyLong/1 -> [DesiredPwmU], [PwmShift_DutyLong]
  Add4/1 -> Switch/1
  [PwmShiftPtr_RiseShort_du] -> Add7/1
  [PwmShiftPtr_RiseMed_du] -> Add7/2
  [PwmShiftPtr_RiseLong] -> Switch/3
  Add34/1 -> Add11/2
  Bus Selector1/3 -> [PwmShiftPtr_RiseShort_du]  "<PwmShiftPtr_RiseShort>"
  [PwmShiftPtr_RiseLong] -> Add3/2
  [DesiredPwmW] -> Add11/1
  Add7/1 -> Relational Operator2/1
  [PwmShift_DutyLong_lo] -> Add27/2
  Constant8/1 -> Bus Creator/1  "PwmShiftPtr_RiseLong"
  Add6/1 -> Bus Creator/3  "PwmShiftPtr_RiseShort"
  [PwmShift_DutyLong] -> Relational Operator7/1
  Add11/1 -> u16TickShiftW/1
  [PwmShiftPtr_RiseLong_du] -> Relational Operator1/1
  Constant7/1 -> Relational Operator1/2
  Add26/1 -> Add9/2
  [PwmShiftPtr_RiseMed] -> Bus Creator1/2  "PwmShiftPtr_RiseMed"
  [PwmShiftPtr_RiseShort] -> Bus Creator1/3  "PwmShiftPtr_RiseShort"
  Add28/1 -> Add10/2
  [DesiredPwmV] -> Add9/1
  Add24/1 -> Add25/2
  [PwmShift_DutyMed] -> Add23/1
  Add22/1 -> Add23/2
  Add29/1 -> Add32/1, Add30/1, Add27/1
  Constant5/1 -> Relational Operator/2
  [PwmShift_DutyShort] -> Add25/1
  [PwmShiftPtr_RiseMed] -> Add4/1
  Bus Selector1/1 -> PwmShiftRiseLong/1, [PwmShiftPtr_RiseLong_du1]  "<PwmShiftPtr_RiseLong>"
  [PwmShift_DutyMed_lo] -> Add30/2
  Constant10/1 -> Add8/1
  Add23/1 -> Bus Creator6/2  "PwmShift_DutyMed"
  Add9/1 -> u16TickShiftV/1
  [PwmShiftPtr_RiseMed_du] -> Add8/2
  Bus Creator1/1 -> Switch1/3
  Constant21/1 -> Bus Creator6/1  "PwmShift_DutyLong"
  Constant19/1 -> Relational Operator7/2
  [PwmShift_DutyLong] -> Bus Creator5/1  "PwmShift_DutyLong"
  Add8/1 -> Switch2/1
  [PwmShift_DutyMed] -> Bus Creator5/2  "PwmShift_DutyMed"
  Bus Creator5/1 -> Switch7/3
  [PwmShift_DutyShort] -> Bus Creator5/3  "PwmShift_DutyShort"
  Add27/1 -> Switch8/3, Relational Operator8/1
  Constant23/1 -> Relational Operator8/2
  Relational Operator2/1 -> Switch2/2
  [PwmShiftPtr_RiseShort_du] -> Switch2/3
  Relational Operator/1 -> Switch/2
  Switch1/1 -> Bus Selector1/1
  Bus Creator6/1 -> Switch7/1
  Relational Operator7/1 -> Switch7/2
  Constant24/1 -> Switch8/1
  Relational Operator8/1 -> Switch8/2
  Switch2/1 -> [PwmShiftPtr_RiseShort_du1]
  Switch/1 -> [PwmShiftPtr_RiseLong_du]
  Bus Selector1/2 -> PwmShiftRiseMed/1, [PwmShiftPtr_RiseMed_du]  "<PwmShiftPtr_RiseMed>"
  Switch7/1 -> Bus Selector2/1
  Switch8/1 -> Bus Creator7/1  "PwmShift_DutyLong"
  Constant25/1 -> Relational Operator9/1
  [PwmShift_DutyMed_lo] -> Relational Operator9/2
  [PwmShift_DutyLong_lo] -> Bus Creator8/1
  Bus Selector/2 -> Add1/2  "<PwmShift_DutyMed>"
  [PwmShift_DutyMed_lo] -> Bus Creator8/2
  [PwmShift_DutyShort_lo] -> Bus Creator8/3
  Bus Selector2/1 -> [PwmShift_DutyLong_lo]  "<PwmShift_DutyLong>"
  Bus Selector2/2 -> [PwmShift_DutyMed_lo]  "<PwmShift_DutyMed>"
  Bus Selector2/3 -> [PwmShift_DutyShort_lo]  "<PwmShift_DutyShort>"
  Relational Operator9/1 -> Switch9/2
  Bus Creator8/1 -> Switch9/3
  Switch9/1 -> Bus Selector/1
  Constant3/1 -> Add1/1
  Constant4/1 -> Add2/1
  Bus Selector/1 -> Add/2  "<PwmShift_DutyLong>"
  Bus Selector/3 -> Add2/2  "<PwmShift_DutyShort>"
  Constant/1 -> Add/1
  Add1/1 -> [PwmShiftPtr_RiseMed]
  Add2/1 -> [PwmShiftPtr_RiseShort]
  Add/1 -> [PwmShiftPtr_RiseLong]

== system Foc/FieldOrientedControl/CurrentControl/MOTOR_STATE_ALIGNMENT/SetPiController/PiCtrl_Calc_D/PiControl ==
  s16InRef : Inport  OutDataTypeStr=int16
  s16InMeas : Inport  Port=2  OutDataTypeStr=int16
  s16Ki : Inport  Port=3  OutDataTypeStr=int16
  s16OutMax : Inport  Port=4  OutDataTypeStr=int16
  s8FacKi : Inport  Port=5  OutDataTypeStr=int8
  s16OutMin : Inport  Port=6  OutDataTypeStr=int16
  s16Kp : Inport  Port=7  OutDataTypeStr=int16
  s8FacKp : Inport  Port=8  OutDataTypeStr=int8
  Add : Sum  Inputs=+-
  Add1 : Sum
  Add2 : Sum
  Data Type Conversion{,1..2,4,7} (5 alike) : DataTypeConversion  OutDataTypeStr=int32  SaturateOnIntegerOverflow=off  RndMeth=Floor
  Data Type Conversion{3,5..6,8} (4 alike) : DataTypeConversion  OutDataTypeStr=uint8  SaturateOnIntegerOverflow=off  RndMeth=Floor
  Data Type Conversion9 : DataTypeConversion  OutDataTypeStr=int16  SaturateOnIntegerOverflow=off  RndMeth=Floor
  Divide : Product  Inputs=**
  Divide1 : Product  Inputs=**
  Relational Operator : RelationalOperator  Operator=>  OutDataTypeStr=boolean  RndMeth=Simplest  InputSameDT=off
  Relational Operator1 : RelationalOperator  Operator=<  OutDataTypeStr=boolean  RndMeth=Simplest  InputSameDT=off
  Relational Operator2 : RelationalOperator  Operator=>  OutDataTypeStr=boolean  RndMeth=Simplest  InputSameDT=off
  Relational Operator3 : RelationalOperator  Operator=<  OutDataTypeStr=boolean  RndMeth=Simplest  InputSameDT=off
  Shift Arithmetic : ArithShift  BitShiftNumberSource=Input port  BitShiftNumber=8  BitShiftDirection=Left
      settings: InputPortMap=u0,p1
  Shift Arithmetic1 : ArithShift  BitShiftNumberSource=Input port  BitShiftNumber=8  BitShiftDirection=Left
      settings: InputPortMap=u0,p1
  Shift Arithmetic2 : ArithShift  BitShiftNumberSource=Input port  BitShiftNumber=8  BitShiftDirection=Right
      settings: InputPortMap=u0,p1
  Shift Arithmetic3 : ArithShift  BitShiftNumberSource=Input port  BitShiftNumber=8  BitShiftDirection=Right
      settings: InputPortMap=u0,p1
  Switch{,1..3} (4 alike) : Switch  Criteria=u2 > Threshold  SaturateOnIntegerOverflow=off  InputSameDT=off
  Unit Delay : UnitDelay  SampleTime=-1  HasFrameUpgradeWarning=on
  s16OutMax1 : InportShadow  Port=4  OutDataTypeStr=int16
  s16OutMax2 : InportShadow  Port=4  OutDataTypeStr=int16
  s16OutMin1 : InportShadow  Port=6  OutDataTypeStr=int16
  s16OutMin2 : InportShadow  Port=6  OutDataTypeStr=int16
  s8FacKi1 : InportShadow  Port=5  OutDataTypeStr=int8
  s8FacKi3 : InportShadow  Port=5  OutDataTypeStr=int8
  s16Out : Outport  OutDataTypeStr=int16
  wires:
  s16OutMin2/1 -> Switch3/1
  s16InRef/1 -> Add/1
  Data Type Conversion7/1 -> Divide1/2
  Add/1 -> Data Type Conversion/1  "s16Err"
  s8FacKi1/1 -> Data Type Conversion5/1
  s16InMeas/1 -> Add/2
  s16Kp/1 -> Data Type Conversion7/1
  s8FacKi3/1 -> Data Type Conversion6/1
  s16Ki/1 -> Data Type Conversion1/1
  s8FacKp/1 -> Data Type Conversion8/1
  Data Type Conversion/1 -> Divide1/1, Divide/1
  Data Type Conversion1/1 -> Divide/2
  s16OutMin/1 -> Data Type Conversion4/1
  Unit Delay/1 -> Add1/2
  Divide1/1 -> Shift Arithmetic3/1
  Data Type Conversion8/1 -> Shift Arithmetic3/2
  s16OutMax/1 -> Data Type Conversion2/1
  s8FacKi/1 -> Data Type Conversion3/1
  Divide/1 -> Add1/1
  Data Type Conversion4/1 -> Shift Arithmetic1/1
  Data Type Conversion5/1 -> Shift Arithmetic1/2
  Shift Arithmetic3/1 -> Add2/1
  Data Type Conversion2/1 -> Shift Arithmetic/1
  Data Type Conversion3/1 -> Shift Arithmetic/2
  Add1/1 -> Switch1/3, Relational Operator/1, Unit Delay/1, Relational Operator1/1  "s32Sum"
  Shift Arithmetic1/1 -> Switch1/1, Relational Operator1/2
  Shift Arithmetic/1 -> Switch/1, Relational Operator/2
  Relational Operator1/1 -> Switch1/2
  Relational Operator/1 -> Switch/2
  Switch1/1 -> Switch/3
  Switch/1 -> Shift Arithmetic2/1
  Data Type Conversion6/1 -> Shift Arithmetic2/2
  Shift Arithmetic2/1 -> Add2/2
  s16OutMax1/1 -> Relational Operator2/2
  Add2/1 -> Data Type Conversion9/1, Relational Operator3/1, Relational Operator2/1  "s32UnLim"
  s16OutMin1/1 -> Relational Operator3/2
  Relational Operator2/1 -> Switch2/2
  Relational Operator3/1 -> Switch3/2
  Data Type Conversion9/1 -> Switch3/3
  s16OutMax2/1 -> Switch2/1
  Switch3/1 -> Switch2/3
  Switch2/1 -> s16Out/1

== system Foc/FieldOrientedControl/CurrentControl/MOTOR_STATE_ALIGNMENT/SetPiController/PiCtrl_Calc_q/PiControl ==
  s16InRef : Inport  OutDataTypeStr=int16
  s16InMeas : Inport  Port=2  OutDataTypeStr=int16
  s16Ki : Inport  Port=3  OutDataTypeStr=int16
  s16OutMax : Inport  Port=4  OutDataTypeStr=int16
  s8FacKi : Inport  Port=5  OutDataTypeStr=int8
  s16OutMin : Inport  Port=6  OutDataTypeStr=int16
  s16Kp : Inport  Port=7  OutDataTypeStr=int16
  s8FacKp : Inport  Port=8  OutDataTypeStr=int8
  Add : Sum  Inputs=+-
  Add1 : Sum
  Add2 : Sum
  Data Type Conversion{,1..2,4,7} (5 alike) : DataTypeConversion  OutDataTypeStr=int32  SaturateOnIntegerOverflow=off  RndMeth=Floor
  Data Type Conversion{3,5..6,8} (4 alike) : DataTypeConversion  OutDataTypeStr=uint8  SaturateOnIntegerOverflow=off  RndMeth=Floor
  Data Type Conversion9 : DataTypeConversion  OutDataTypeStr=int16  SaturateOnIntegerOverflow=off  RndMeth=Floor
  Divide : Product  Inputs=**
  Divide1 : Product  Inputs=**
  Relational Operator : RelationalOperator  Operator=>  OutDataTypeStr=boolean  RndMeth=Simplest  InputSameDT=off
  Relational Operator1 : RelationalOperator  Operator=<  OutDataTypeStr=boolean  RndMeth=Simplest  InputSameDT=off
  Relational Operator2 : RelationalOperator  Operator=>  OutDataTypeStr=boolean  RndMeth=Simplest  InputSameDT=off
  Relational Operator3 : RelationalOperator  Operator=<  OutDataTypeStr=boolean  RndMeth=Simplest  InputSameDT=off
  Shift Arithmetic : ArithShift  BitShiftNumberSource=Input port  BitShiftNumber=8  BitShiftDirection=Left
      settings: InputPortMap=u0,p1
  Shift Arithmetic1 : ArithShift  BitShiftNumberSource=Input port  BitShiftNumber=8  BitShiftDirection=Left
      settings: InputPortMap=u0,p1
  Shift Arithmetic2 : ArithShift  BitShiftNumberSource=Input port  BitShiftNumber=8  BitShiftDirection=Right
      settings: InputPortMap=u0,p1
  Shift Arithmetic3 : ArithShift  BitShiftNumberSource=Input port  BitShiftNumber=8  BitShiftDirection=Right
      settings: InputPortMap=u0,p1
  Switch{,1..3} (4 alike) : Switch  Criteria=u2 > Threshold  SaturateOnIntegerOverflow=off  InputSameDT=off
  Unit Delay : UnitDelay  SampleTime=-1  HasFrameUpgradeWarning=on
  s16OutMax1 : InportShadow  Port=4  OutDataTypeStr=int16
  s16OutMax2 : InportShadow  Port=4  OutDataTypeStr=int16
  s16OutMin1 : InportShadow  Port=6  OutDataTypeStr=int16
  s16OutMin2 : InportShadow  Port=6  OutDataTypeStr=int16
  s8FacKi1 : InportShadow  Port=5  OutDataTypeStr=int8
  s8FacKi3 : InportShadow  Port=5  OutDataTypeStr=int8
  s16Out : Outport  OutDataTypeStr=int16
  wires:
  s16OutMin2/1 -> Switch3/1
  s16InRef/1 -> Add/1
  Data Type Conversion7/1 -> Divide1/2
  Add/1 -> Data Type Conversion/1  "s16Err"
  s8FacKi1/1 -> Data Type Conversion5/1
  s16InMeas/1 -> Add/2
  s16Kp/1 -> Data Type Conversion7/1
  s8FacKi3/1 -> Data Type Conversion6/1
  s16Ki/1 -> Data Type Conversion1/1
  s8FacKp/1 -> Data Type Conversion8/1
  Data Type Conversion/1 -> Divide1/1, Divide/1
  Data Type Conversion1/1 -> Divide/2
  s16OutMin/1 -> Data Type Conversion4/1
  Unit Delay/1 -> Add1/2
  Divide1/1 -> Shift Arithmetic3/1
  Data Type Conversion8/1 -> Shift Arithmetic3/2
  s16OutMax/1 -> Data Type Conversion2/1
  s8FacKi/1 -> Data Type Conversion3/1
  Divide/1 -> Add1/1
  Data Type Conversion4/1 -> Shift Arithmetic1/1
  Data Type Conversion5/1 -> Shift Arithmetic1/2
  Shift Arithmetic3/1 -> Add2/1
  Data Type Conversion2/1 -> Shift Arithmetic/1
  Data Type Conversion3/1 -> Shift Arithmetic/2
  Add1/1 -> Unit Delay/1, Switch1/3, Relational Operator/1, Relational Operator1/1  "s32Sum"
  Shift Arithmetic1/1 -> Relational Operator1/2, Switch1/1
  Shift Arithmetic/1 -> Switch/1, Relational Operator/2
  Relational Operator1/1 -> Switch1/2
  Relational Operator/1 -> Switch/2
  Switch1/1 -> Switch/3
  Switch/1 -> Shift Arithmetic2/1
  Data Type Conversion6/1 -> Shift Arithmetic2/2
  Shift Arithmetic2/1 -> Add2/2
  s16OutMax1/1 -> Relational Operator2/2
  Add2/1 -> Data Type Conversion9/1, Relational Operator3/1, Relational Operator2/1  "s32UnLim"
  s16OutMin1/1 -> Relational Operator3/2
  Relational Operator2/1 -> Switch2/2
  Relational Operator3/1 -> Switch3/2
  Data Type Conversion9/1 -> Switch3/3
  s16OutMax2/1 -> Switch2/1
  Switch3/1 -> Switch2/3
  Switch2/1 -> s16Out/1

== system Foc/FieldOrientedControl/CurrentControl/MOTOR_STATE_BRAKE/SetPiController/PiCtrl_Calc_D/PiControl ==
  s16InRef : Inport  OutDataTypeStr=int16
  s16InMeas : Inport  Port=2  OutDataTypeStr=int16
  s16Ki : Inport  Port=3  OutDataTypeStr=int16
  s16OutMax : Inport  Port=4  OutDataTypeStr=int16
  s8FacKi : Inport  Port=5  OutDataTypeStr=int8
  s16OutMin : Inport  Port=6  OutDataTypeStr=int16
  s16Kp : Inport  Port=7  OutDataTypeStr=int16
  s8FacKp : Inport  Port=8  OutDataTypeStr=int8
  Add : Sum  Inputs=+-
  Add1 : Sum
  Add2 : Sum
  Data Type Conversion{,1..2,4,7} (5 alike) : DataTypeConversion  OutDataTypeStr=int32  SaturateOnIntegerOverflow=off  RndMeth=Floor
  Data Type Conversion{3,5..6,8} (4 alike) : DataTypeConversion  OutDataTypeStr=uint8  SaturateOnIntegerOverflow=off  RndMeth=Floor
  Data Type Conversion9 : DataTypeConversion  OutDataTypeStr=int16  SaturateOnIntegerOverflow=off  RndMeth=Floor
  Divide : Product  Inputs=**
  Divide1 : Product  Inputs=**
  Relational Operator : RelationalOperator  Operator=>  OutDataTypeStr=boolean  RndMeth=Simplest  InputSameDT=off
  Relational Operator1 : RelationalOperator  Operator=<  OutDataTypeStr=boolean  RndMeth=Simplest  InputSameDT=off
  Relational Operator2 : RelationalOperator  Operator=>  OutDataTypeStr=boolean  RndMeth=Simplest  InputSameDT=off
  Relational Operator3 : RelationalOperator  Operator=<  OutDataTypeStr=boolean  RndMeth=Simplest  InputSameDT=off
  Shift Arithmetic : ArithShift  BitShiftNumberSource=Input port  BitShiftNumber=8  BitShiftDirection=Left
      settings: InputPortMap=u0,p1
  Shift Arithmetic1 : ArithShift  BitShiftNumberSource=Input port  BitShiftNumber=8  BitShiftDirection=Left
      settings: InputPortMap=u0,p1
  Shift Arithmetic2 : ArithShift  BitShiftNumberSource=Input port  BitShiftNumber=8  BitShiftDirection=Right
      settings: InputPortMap=u0,p1
  Shift Arithmetic3 : ArithShift  BitShiftNumberSource=Input port  BitShiftNumber=8  BitShiftDirection=Right
      settings: InputPortMap=u0,p1
  Switch{,1..3} (4 alike) : Switch  Criteria=u2 > Threshold  SaturateOnIntegerOverflow=off  InputSameDT=off
  Unit Delay : UnitDelay  SampleTime=-1  HasFrameUpgradeWarning=on
  s16OutMax1 : InportShadow  Port=4  OutDataTypeStr=int16
  s16OutMax2 : InportShadow  Port=4  OutDataTypeStr=int16
  s16OutMin1 : InportShadow  Port=6  OutDataTypeStr=int16
  s16OutMin2 : InportShadow  Port=6  OutDataTypeStr=int16
  s8FacKi1 : InportShadow  Port=5  OutDataTypeStr=int8
  s8FacKi3 : InportShadow  Port=5  OutDataTypeStr=int8
  s16Out : Outport  OutDataTypeStr=int16
  wires:
  s16OutMin2/1 -> Switch3/1
  s16InRef/1 -> Add/1
  Data Type Conversion7/1 -> Divide1/2
  Add/1 -> Data Type Conversion/1  "s16Err"
  s8FacKi1/1 -> Data Type Conversion5/1
  s16InMeas/1 -> Add/2
  s16Kp/1 -> Data Type Conversion7/1
  s8FacKi3/1 -> Data Type Conversion6/1
  s16Ki/1 -> Data Type Conversion1/1
  s8FacKp/1 -> Data Type Conversion8/1
  Data Type Conversion/1 -> Divide/1, Divide1/1
  Data Type Conversion1/1 -> Divide/2
  s16OutMin/1 -> Data Type Conversion4/1
  Unit Delay/1 -> Add1/2
  Divide1/1 -> Shift Arithmetic3/1
  Data Type Conversion8/1 -> Shift Arithmetic3/2
  s16OutMax/1 -> Data Type Conversion2/1
  s8FacKi/1 -> Data Type Conversion3/1
  Divide/1 -> Add1/1
  Data Type Conversion4/1 -> Shift Arithmetic1/1
  Data Type Conversion5/1 -> Shift Arithmetic1/2
  Shift Arithmetic3/1 -> Add2/1
  Data Type Conversion2/1 -> Shift Arithmetic/1
  Data Type Conversion3/1 -> Shift Arithmetic/2
  Add1/1 -> Relational Operator/1, Switch1/3, Unit Delay/1, Relational Operator1/1  "s32Sum"
  Shift Arithmetic1/1 -> Switch1/1, Relational Operator1/2
  Shift Arithmetic/1 -> Switch/1, Relational Operator/2
  Relational Operator1/1 -> Switch1/2
  Relational Operator/1 -> Switch/2
  Switch1/1 -> Switch/3
  Switch/1 -> Shift Arithmetic2/1
  Data Type Conversion6/1 -> Shift Arithmetic2/2
  Shift Arithmetic2/1 -> Add2/2
  s16OutMax1/1 -> Relational Operator2/2
  Add2/1 -> Relational Operator3/1, Data Type Conversion9/1, Relational Operator2/1  "s32UnLim"
  s16OutMin1/1 -> Relational Operator3/2
  Relational Operator2/1 -> Switch2/2
  Relational Operator3/1 -> Switch3/2
  Data Type Conversion9/1 -> Switch3/3
  s16OutMax2/1 -> Switch2/1
  Switch3/1 -> Switch2/3
  Switch2/1 -> s16Out/1

== system Foc/FieldOrientedControl/CurrentControl/MOTOR_STATE_BRAKE/SetPiController/PiCtrl_Calc_q/PiControl ==
  s16InRef : Inport  OutDataTypeStr=int16
  s16InMeas : Inport  Port=2  OutDataTypeStr=int16
  s16Ki : Inport  Port=3  OutDataTypeStr=int16
  s16OutMax : Inport  Port=4  OutDataTypeStr=int16
  s8FacKi : Inport  Port=5  OutDataTypeStr=int8
  s16OutMin : Inport  Port=6  OutDataTypeStr=int16
  s16Kp : Inport  Port=7  OutDataTypeStr=int16
  s8FacKp : Inport  Port=8  OutDataTypeStr=int8
  Add : Sum  Inputs=+-
  Add1 : Sum
  Add2 : Sum
  Data Type Conversion{,1..2,4,7} (5 alike) : DataTypeConversion  OutDataTypeStr=int32  SaturateOnIntegerOverflow=off  RndMeth=Floor
  Data Type Conversion{3,5..6,8} (4 alike) : DataTypeConversion  OutDataTypeStr=uint8  SaturateOnIntegerOverflow=off  RndMeth=Floor
  Data Type Conversion9 : DataTypeConversion  OutDataTypeStr=int16  SaturateOnIntegerOverflow=off  RndMeth=Floor
  Divide : Product  Inputs=**
  Divide1 : Product  Inputs=**
  Relational Operator : RelationalOperator  Operator=>  OutDataTypeStr=boolean  RndMeth=Simplest  InputSameDT=off
  Relational Operator1 : RelationalOperator  Operator=<  OutDataTypeStr=boolean  RndMeth=Simplest  InputSameDT=off
  Relational Operator2 : RelationalOperator  Operator=>  OutDataTypeStr=boolean  RndMeth=Simplest  InputSameDT=off
  Relational Operator3 : RelationalOperator  Operator=<  OutDataTypeStr=boolean  RndMeth=Simplest  InputSameDT=off
  Shift Arithmetic : ArithShift  BitShiftNumberSource=Input port  BitShiftNumber=8  BitShiftDirection=Left
      settings: InputPortMap=u0,p1
  Shift Arithmetic1 : ArithShift  BitShiftNumberSource=Input port  BitShiftNumber=8  BitShiftDirection=Left
      settings: InputPortMap=u0,p1
  Shift Arithmetic2 : ArithShift  BitShiftNumberSource=Input port  BitShiftNumber=8  BitShiftDirection=Right
      settings: InputPortMap=u0,p1
  Shift Arithmetic3 : ArithShift  BitShiftNumberSource=Input port  BitShiftNumber=8  BitShiftDirection=Right
      settings: InputPortMap=u0,p1
  Switch{,1..3} (4 alike) : Switch  Criteria=u2 > Threshold  SaturateOnIntegerOverflow=off  InputSameDT=off
  Unit Delay : UnitDelay  SampleTime=-1  HasFrameUpgradeWarning=on
  s16OutMax1 : InportShadow  Port=4  OutDataTypeStr=int16
  s16OutMax2 : InportShadow  Port=4  OutDataTypeStr=int16
  s16OutMin1 : InportShadow  Port=6  OutDataTypeStr=int16
  s16OutMin2 : InportShadow  Port=6  OutDataTypeStr=int16
  s8FacKi1 : InportShadow  Port=5  OutDataTypeStr=int8
  s8FacKi3 : InportShadow  Port=5  OutDataTypeStr=int8
  s16Out : Outport  OutDataTypeStr=int16
  wires:
  s16OutMin2/1 -> Switch3/1
  s16InRef/1 -> Add/1
  Data Type Conversion7/1 -> Divide1/2
  Add/1 -> Data Type Conversion/1  "s16Err"
  s8FacKi1/1 -> Data Type Conversion5/1
  s16InMeas/1 -> Add/2
  s16Kp/1 -> Data Type Conversion7/1
  s8FacKi3/1 -> Data Type Conversion6/1
  s16Ki/1 -> Data Type Conversion1/1
  s8FacKp/1 -> Data Type Conversion8/1
  Data Type Conversion/1 -> Divide/1, Divide1/1
  Data Type Conversion1/1 -> Divide/2
  s16OutMin/1 -> Data Type Conversion4/1
  Unit Delay/1 -> Add1/2
  Divide1/1 -> Shift Arithmetic3/1
  Data Type Conversion8/1 -> Shift Arithmetic3/2
  s16OutMax/1 -> Data Type Conversion2/1
  s8FacKi/1 -> Data Type Conversion3/1
  Divide/1 -> Add1/1
  Data Type Conversion4/1 -> Shift Arithmetic1/1
  Data Type Conversion5/1 -> Shift Arithmetic1/2
  Shift Arithmetic3/1 -> Add2/1
  Data Type Conversion2/1 -> Shift Arithmetic/1
  Data Type Conversion3/1 -> Shift Arithmetic/2
  Add1/1 -> Unit Delay/1, Switch1/3, Relational Operator/1, Relational Operator1/1  "s32Sum"
  Shift Arithmetic1/1 -> Relational Operator1/2, Switch1/1
  Shift Arithmetic/1 -> Switch/1, Relational Operator/2
  Relational Operator1/1 -> Switch1/2
  Relational Operator/1 -> Switch/2
  Switch1/1 -> Switch/3
  Switch/1 -> Shift Arithmetic2/1
  Data Type Conversion6/1 -> Shift Arithmetic2/2
  Shift Arithmetic2/1 -> Add2/2
  s16OutMax1/1 -> Relational Operator2/2
  Add2/1 -> Data Type Conversion9/1, Relational Operator2/1, Relational Operator3/1  "s32UnLim"
  s16OutMin1/1 -> Relational Operator3/2
  Relational Operator2/1 -> Switch2/2
  Relational Operator3/1 -> Switch3/2
  Data Type Conversion9/1 -> Switch3/3
  s16OutMax2/1 -> Switch2/1
  Switch3/1 -> Switch2/3
  Switch2/1 -> s16Out/1
